simulink model "FOC_Motor_Control"  (R2020b)
settings: Solver=FixedStepDiscrete  StartTime=0.0  StopTime=10.0  FixedStep=Fixed_Step_Size  RelTol=1e-3
values from neighbouring files (symbols this model uses):
  Angle = 1.0    [Hall_Flux_FOC_Data.sldd]    (also in Motor_Control_Data.sldd)
  Cosine_table = 1.0 0.99999529 0.99999058 0.99998587 0.99998116 0.99996704 0.99995291 0.99993885 0.99992472 0.99990118 0.99987763 0.99985409 0.9998306 0.99979764 0.99976468 0.99973178 0.99969882 0.99965644 0.99961412 0.99957174 0.99952942 0.99947762 0.99942589 0.99937415 0.99932235 0.9992612 0.99920005 0.99913889 0.99907768 0.99900717 0.99893659 0.99886602 0.99879545 0.99871546 0.99863547 0.99855554 0.99847555 0.    [Hall_Flux_FOC_Data.sldd]    (also in Motor_Control_Data.sldd)
  Flux = 0.0109    [G474_FOC_LADRC.sldd]    (also in G474_FOC_NONOBSERVER.sldd = 0.0109
  HaLL_AngleShift = -0.25    [Hall_Flux_FOC_Data.sldd]
  HaLL_Sector1 = 5.236    [Hall_Flux_FOC_Data.sldd]
  HaLL_Sector2 = 1.0472    [Hall_Flux_FOC_Data.sldd]
  HaLL_Sector3 = 0.0    [Hall_Flux_FOC_Data.sldd]
  HaLL_Sector4 = 3.1415    [Hall_Flux_FOC_Data.sldd]
  HaLL_Sector5 = 4.1888    [Hall_Flux_FOC_Data.sldd]
  HaLL_Sector6 = 2.0944    [Hall_Flux_FOC_Data.sldd]
  HaLL_Timer_T = 1.0E-5    [Hall_Flux_FOC_Data.sldd]
  ID_Ki = 1.3    [Hall_Flux_FOC_Data.sldd]    (also in Motor_Control_Data.sldd = 48.0
  ID_Kp = 0.4    [Hall_Flux_FOC_Data.sldd]    (also in Motor_Control_Data.sldd = 0.84
  inverter = struct    [PMSM_Parameters.m]
  IQ_Ki = 1.6    [Hall_Flux_FOC_Data.sldd]    (also in Motor_Control_Data.sldd = 48.0
  IQ_Kp = 0.4    [Hall_Flux_FOC_Data.sldd]    (also in Motor_Control_Data.sldd = 1.869
  LADRC_b0 = 10000.0    [G474_FOC_LADRC.sldd]    (also in Hall_Flux_FOC_Data.sldd = 80000.0
  LADRC_Omega_c = 100.0    [G474_FOC_LADRC.sldd]    (also in Hall_Flux_FOC_Data.sldd = 80.0
  Ld = 0.0004    [Hall_Flux_FOC_Data.sldd]    (also in Motor_Control_Data.sldd = 0.00014
  Lq = 0.00045    [Hall_Flux_FOC_Data.sldd]    (also in Motor_Control_Data.sldd = 0.0003115
  OPL_Speed = 800.0    [Hall_Flux_FOC_Data.sldd]
  OPL_Time = 2.0    [Hall_Flux_FOC_Data.sldd]
  OPL_Torque = 3.0    [Hall_Flux_FOC_Data.sldd]
  Over_modulation = 0.0    [Hall_Flux_FOC_Data.sldd]    (also in Motor_Control_Data.sldd)
  pll_omega = 5000.0    [G474_FOC_LADRC.sldd]    (also in G474_FOC_NONOBSERVER.sldd)
  pll_xi = 10.0    [G474_FOC_LADRC.sldd]    (also in G474_FOC_NONOBSERVER.sldd)
  Pole_Pairs = 2.0    [Hall_Flux_FOC_Data.sldd]    (also in Motor_Control_Data.sldd = 4.0
  PWM_Frequency = 10000.0    [Hall_Flux_FOC_Data.sldd]    (also in Motor_Control_Data.sldd = 20000.0
  R = 0.405    [Hall_Flux_FOC_Data.sldd]    (also in Motor_Control_Data.sldd = 0.016
  Sine_table = 0.0 0.0015339879 0.0030679768 0.0046019657 0.0061359555 0.0076698866 0.0092038177 0.010737749 0.012271681 0.013805497 0.015339312 0.016873131 0.018406944 0.019940587 0.021474229 0.023007872 0.024541514 0.026074925 0.027608337 0.029141748 0.03067516 0.032208283 0.033741407 0.035274528 0.036807653 0.038340431 0.039873205 0.04140598 0.042938754 0.04447113 0.046003502 0.047535874 0.049068246 0.0506001    [Hall_Flux_FOC_Data.sldd]    (also in Motor_Control_Data.sldd)
  Speed_Ki = 0.06    [Hall_Flux_FOC_Data.sldd]    (also in Motor_Control_Data.sldd = 10.809
  Speed_Kp = 0.002    [Hall_Flux_FOC_Data.sldd]    (also in Motor_Control_Data.sldd = 0.08
  Speed_PI_OutputMax = 3.0    [Hall_Flux_FOC_Data.sldd]    (also in Motor_Control_Data.sldd = 700.0
  Speed_PI_OutputMin = -5.0    [Hall_Flux_FOC_Data.sldd]    (also in Motor_Control_Data.sldd = -700.0
  SpeedFilter_Fn = 0.3    [Hall_Flux_FOC_Data.sldd]    (also in Motor_Control_Data.sldd = 0.2
  TorqueMode = 0.0    [Hall_Flux_FOC_Data.sldd]    (also in Motor_Control_Data.sldd)
undefined symbols (not defined in the file or in its folder): DiscIntNeverNeededParam, Flux_Gain, Flux_Theta_Enable, magnitude, SVPWM
libraries: simulink x6, dspstat3 x1, pid_lib x1
(part 2 of 3)

== system FOC_Motor_Control/Motor_Control/Motor_Control_Function/FOC_Control_100us/FOC/Inverse_Park_Transform ==
  D : Inport
  Q : Inport  Port=2
  Sin_Coefficient : Inport  Port=3
  Cos_Coefficient : Inport  Port=4
  Theta : Inport  Port=5
  Add : Sum
  Add1 : Sum  Inputs=+-  OutDataTypeStr=Inherit: Same as first input
  Add2 : Sum  OutDataTypeStr=Inherit: Same as first input
  Add3 : Sum
  Cos_Coefficient1 : InportShadow  Port=4
  Harmonic_injection : Subsystem  Commented=on
  Product{1..4} (4 alike) : Product  RndMeth=Simplest  OutDataTypeStr=Inherit: Same as first input
  Scope : Scope  NumInputPorts=2
  Sin_Coefficient1 : InportShadow  Port=3
  Alpha : Outport  VectorParamsAs1DForOutWhenUnconnected=off
  Beta : Outport  Port=2  VectorParamsAs1DForOutWhenUnconnected=off
  wires:
  Product3/1 -> Add2/1
  Product4/1 -> Add2/2
  Product1/1 -> Add1/1
  Product2/1 -> Add1/2
  Cos_Coefficient1/1 -> Product4/2
  Sin_Coefficient/1 -> Product2/2
  D/1 -> Product3/1, Product1/1
  Q/1 -> Product2/1, Product4/1
  Sin_Coefficient1/1 -> Product3/2
  Cos_Coefficient/1 -> Product1/2
  Add1/1 -> Add/1
  Add/1 -> Alpha/1
  Harmonic_injection/1(Out1) -> Scope/1, Add/2
  Add2/1 -> Add3/2
  Add3/1 -> Beta/1
  Harmonic_injection/2(Out2) -> Scope/2, Add3/1
  Theta/1 -> Harmonic_injection/1(Input)

== system FOC_Motor_Control/Motor_Control/Motor_Control_Function/FOC_Control_100us/FOC/Obs_Angle ==
  Obs_Angle : Inport
  Action Port : ActionPort  ActionPortLabel=if(u1==1)
  Out1 : Outport
  wires:
  Obs_Angle/1 -> Out1/1

== system FOC_Motor_Control/Motor_Control/Motor_Control_Function/FOC_Control_100us/FOC/OpenLoop ==
  OPL_Speed : Inport
  OPL_Torque : Inport  Port=2
  OPL_Time : Inport  Port=3
  Action Port : ActionPort  ActionPortLabel=case [ 1 ]:
  2pi2 : Constant  Value=2*pi  OutDataTypeStr=single
  Discrete-Time Integrator1 : DiscreteIntegrator  SampleTime=-1  ICPrevOutput=DiscIntNeverNeededParam  ICPrevScaledInput=DiscIntNeverNeededParam
  Discrete-Time Integrator2 : DiscreteIntegrator  SampleTime=-1  ICPrevOutput=DiscIntNeverNeededParam  ICPrevScaledInput=DiscIntNeverNeededParam
  Mod2 : Math  Operator=mod  SaturateOnIntegerOverflow=on
  Product : Product
  Scope : Scope
  Scope1 : Scope
  We : Gain  Gain=Pole_Pairs*2*pi/60  OutDataTypeStr=single  ParamDataTypeStr=Inherit: Same as input
  Force_Angle : Outport
  OPL_Torque_Com : Outport  Port=2
  wires:
  OPL_Speed/1 -> Product/1
  Product/1 -> Discrete-Time Integrator2/1
  Discrete-Time Integrator1/1 -> Mod2/1
  Discrete-Time Integrator2/1 -> Scope/1, We/1
  We/1 -> Discrete-Time Integrator1/1  "Delta_Theta"
  Mod2/1 -> Force_Angle/1, Scope1/1
  OPL_Torque/1 -> OPL_Torque_Com/1
  OPL_Time/1 -> Product/2
  2pi2/1 -> Mod2/2

== system FOC_Motor_Control/Motor_Control/Motor_Control_Function/FOC_Control_100us/FOC/Park_Transform ==
  Alpha : Inport
  Beta : Inport  Port=2
  Sin_Coefficient : Inport  Port=3
  Cos_Coefficient : Inport  Port=4
  Add1 : Sum  OutDataTypeStr=Inherit: Same as first input
  Add2 : Sum  Inputs=-+  OutDataTypeStr=Inherit: Same as first input
  Alpha1 : InportShadow
  Beta1 : InportShadow  Port=2
  Cos_Coefficient1 : InportShadow  Port=4
  Produc3t : Product  RndMeth=Simplest  OutDataTypeStr=Inherit: Same as first input
  Product1 : Product  RndMeth=Simplest  OutDataTypeStr=Inherit: Same as first input
  Product2 : Product  RndMeth=Simplest  OutDataTypeStr=Inherit: Same as first input
  Product4 : Product  RndMeth=Simplest  OutDataTypeStr=Inherit: Same as first input
  Sin_Coefficient1 : InportShadow  Port=3
  D : Outport  VectorParamsAs1DForOutWhenUnconnected=off
  Q : Outport  Port=2  VectorParamsAs1DForOutWhenUnconnected=off
  wires:
  Produc3t/1 -> Add2/1
  Product4/1 -> Add2/2
  Product1/1 -> Add1/1
  Product2/1 -> Add1/2
  Alpha1/1 -> Produc3t/1
  Sin_Coefficient1/1 -> Produc3t/2
  Cos_Coefficient1/1 -> Product4/2
  Beta1/1 -> Product4/1
  Alpha/1 -> Product1/1
  Cos_Coefficient/1 -> Product1/2
  Beta/1 -> Product2/1
  Sin_Coefficient/1 -> Product2/2
  Add1/1 -> D/1
  Add2/1 -> Q/1

== system FOC_Motor_Control/Motor_Control/Motor_Control_Function/FOC_Control_100us/FOC/Q_Current_PI ==
  Reset : Inport
  Bus_voltage : Inport  Port=2
  Current_Command : Inport  Port=3
  Current_Measured : Inport  Port=4
  Add2 : Sum  Inputs=|+-
  IQ_Control : Subsystem
  Vq_voltage : Outport  VectorParamsAs1DForOutWhenUnconnected=off
  wires:
  Current_Command/1 -> Add2/1
  Current_Measured/1 -> Add2/2
  Add2/1 -> IQ_Control/3(Err)  "currentControlError"
  Reset/1 -> IQ_Control/1(Reset)
  Bus_voltage/1 -> IQ_Control/2(Bus_voltage)
  IQ_Control/1(PI_Out) -> Vq_voltage/1

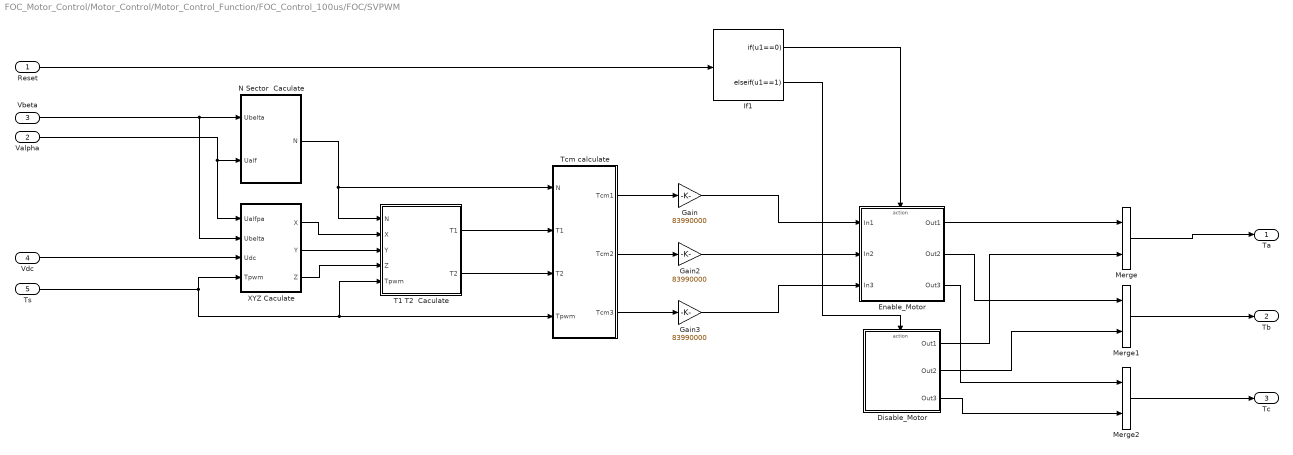
== system FOC_Motor_Control/Motor_Control/Motor_Control_Function/FOC_Control_100us/FOC/SVPWM ==
  Reset : Inport
  Valpha : Inport  Port=2
  Vbeta : Inport  Port=3
  Vdc : Inport  Port=4
  Ts : Inport  Port=5
  Disable_Motor : Subsystem  TreatAsAtomicUnit=on
  Enable_Motor : Subsystem  TreatAsAtomicUnit=on
  Gain : Gain  Gain=83990000
  Gain2 : Gain  Gain=83990000
  Gain3 : Gain  Gain=83990000
  If1 : If  IfExpression=u1==0  ElseIfExpressions=u1==1  ShowElse=off
  Merge : Merge
  Merge1 : Merge
  Merge2 : Merge
  N Sector  Caculate : Subsystem  TreatAsAtomicUnit=on
  T1 T2  Caculate : Subsystem  TreatAsAtomicUnit=on
  Tcm calculate : Subsystem  TreatAsAtomicUnit=on
  XYZ Caculate : Subsystem  TreatAsAtomicUnit=on
  Ta : Outport
  Tb : Outport  Port=2
  Tc : Outport  Port=3
  wires:
  T1 T2  Caculate/2(T2) -> Tcm calculate/3(T2)
  XYZ Caculate/1(X) -> T1 T2  Caculate/2(X)
  N Sector  Caculate/1(N) -> T1 T2  Caculate/1(N), Tcm calculate/1(N)
  Vdc/1 -> XYZ Caculate/3(Udc)
  T1 T2  Caculate/1(T1) -> Tcm calculate/2(T1)
  XYZ Caculate/3(Z) -> T1 T2  Caculate/4(Z)
  XYZ Caculate/2(Y) -> T1 T2  Caculate/3(Y)
  Valpha/1 -> N Sector  Caculate/2(Ualf), XYZ Caculate/1(Ualfpa)
  Vbeta/1 -> N Sector  Caculate/1(Ubelta), XYZ Caculate/2(Ubelta)
  Ts/1 -> T1 T2  Caculate/5(Tpwm), Tcm calculate/4(Tpwm), XYZ Caculate/4(Tpwm)
  Gain/1 -> Enable_Motor/1(In1)
  Gain2/1 -> Enable_Motor/2(In2)
  Reset/1 -> If1/1
  If1/1 -> Enable_Motor/Action
  If1/2 -> Disable_Motor/Action
  Gain3/1 -> Enable_Motor/3(In3)
  Enable_Motor/1(Out1) -> Merge/1
  Disable_Motor/1(Out1) -> Merge/2
  Enable_Motor/2(Out2) -> Merge1/1
  Disable_Motor/2(Out2) -> Merge1/2
  Enable_Motor/3(Out3) -> Merge2/1
  Disable_Motor/3(Out3) -> Merge2/2
  Merge/1 -> Ta/1
  Merge1/1 -> Tb/1
  Merge2/1 -> Tc/1
  Tcm calculate/1(Tcm1) -> Gain/1
  Tcm calculate/2(Tcm2) -> Gain2/1
  Tcm calculate/3(Tcm3) -> Gain3/1

== system FOC_Motor_Control/Motor_Control/Motor_Control_Function/FOC_Control_100us/FOC/Sine_Cosine ==
  note: Sine Cosine Coefficients
  P : Inport
  Cosine : Lookup_n-D  NumberOfTableDimensions=1  LookupTableObject=''  BreakpointsForDimension1=[0:2*pi/4095:2*pi]  BreakpointsForDimension1FirstPoint=10  BreakpointsForDimension2FirstPoint=10  BreakpointsForDimension1Spacing=12  BreakpointsForDimension2Spacing=12  IndexSearchMethod=Evenly spaced points  Table=Cosine_table  InterpMethod=Flat  DiagnosticForOutOfRangeInput=Error  InternalRulePriority=Speed  RndMeth=Simplest  InputSameDT=on
  Saturation : Saturate  UpperLimit=2*pi-0.0001  LowerLimit=0+0.0001
  Scope : Scope  NumInputPorts=2
  Sine : Lookup_n-D  NumberOfTableDimensions=1  LookupTableObject=''  BreakpointsForDimension1=[0:2*pi/4095:2*pi]  BreakpointsForDimension1FirstPoint=10  BreakpointsForDimension2FirstPoint=10  BreakpointsForDimension1Spacing=12  BreakpointsForDimension2Spacing=12  IndexSearchMethod=Evenly spaced points  Table=Sine_table  InterpMethod=Flat  DiagnosticForOutOfRangeInput=Error  InternalRulePriority=Speed  RndMeth=Simplest  InputSameDT=on
  Sin : Outport  VectorParamsAs1DForOutWhenUnconnected=off
  Cos : Outport  Port=2  VectorParamsAs1DForOutWhenUnconnected=off
  wires:
  P/1 -> Saturation/1  "position"
  Sine/1 -> Scope/1, Sin/1
  Cosine/1 -> Scope/2, Cos/1
  Saturation/1 -> Cosine/1, Sine/1

== system FOC_Motor_Control/Motor_Control/Motor_Control_Function/FOC_Control_100us/FOC/Subsystem ==
  In1 : Inport
  In2 : Inport  Port=2
  Action Port : ActionPort  ActionPortLabel=case [ 2 ]:
  Out1 : Outport
  Out2 : Outport  Port=2
  wires:
  In1/1 -> Out1/1
  In2/1 -> Out2/1

== system FOC_Motor_Control/Motor_Control/Motor_Control_Function/Angle_Speed_100us/SpeedAndAngle/ACC_OMG/LPF ==
  u : Inport
  Add : Sum  Inputs=+-
  Add1 : Sum
  Constant1 : Constant  Value=SpeedFilter_Fn  OutDataTypeStr=single
  Divide1 : Product  Inputs=**
  Unit Delay : UnitDelay  SampleTime=-1  HasFrameUpgradeWarning=on
  y : Outport
  wires:
  Constant1/1 -> Divide1/1
  u/1 -> Add/1
  Add/1 -> Divide1/2
  Divide1/1 -> Add1/1
  Unit Delay/1 -> Add/2, Add1/2
  Add1/1 -> Unit Delay/1, y/1

== system FOC_Motor_Control/Motor_Control/Motor_Control_Function/Angle_Speed_100us/SpeedAndAngle/ACC_OMG/Six_point ==
  In1 : Inport
  Merge2 : Merge  Inputs=6
  Scope : Scope  NumInputPorts=2
  Sector_1 : Subsystem
  Sector_2 : Subsystem
  Sector_3 : Subsystem
  Sector_4 : Subsystem
  Sector_5 : Subsystem
  Sector_6 : Subsystem
  Switch Case2 : SwitchCase  CaseConditions={1,2,3,4,5,6}  ShowDefaultCase=off
  Out1 : Outport
  wires:
  Sector_4/1(Angle_0) -> Merge2/4
  Switch Case2/5 -> Sector_5/Action
  Sector_6/1(Angle_0) -> Merge2/6
  Sector_5/1(Angle_0) -> Merge2/5
  Switch Case2/6 -> Sector_6/Action
  Switch Case2/3 -> Sector_3/Action
  Switch Case2/4 -> Sector_4/Action
  Sector_1/1(Angle_0) -> Merge2/1
  Switch Case2/2 -> Sector_2/Action
  In1/1 -> Scope/1, Switch Case2/1
  Sector_3/1(Angle_0) -> Merge2/3
  Switch Case2/1 -> Sector_1/Action
  Sector_2/1(Angle_0) -> Merge2/2
  Merge2/1 -> Scope/2, Out1/1

== system FOC_Motor_Control/Motor_Control/Motor_Control_Function/Angle_Speed_100us/SpeedAndAngle/ADC_IRQ/HallAngle_calibration ==
  Angle_input : Inport
  Angle_offset : Constant  Value=HaLL_AngleShift
  If Action Subsystem1 : Subsystem  TreatAsAtomicUnit=on
  If Action Subsystem2 : Subsystem  TreatAsAtomicUnit=on
  If Action Subsystem3 : Subsystem  TreatAsAtomicUnit=on
  If1 : If  IfExpression=u1 > 6.283185307  ElseIfExpressions=u1<0
  Merge1 : Merge  Inputs=3
  Subtract1 : Sum
  Angle_output : Outport
  wires:
  Angle_input/1 -> Subtract1/1
  Angle_offset/1 -> Subtract1/2  "Control_ModeCommand"
  If1/1 -> If Action Subsystem2/Action
  If1/3 -> If Action Subsystem1/Action
  If Action Subsystem2/1(Out1) -> Merge1/1
  Subtract1/1 -> If Action Subsystem3/1(In1), If Action Subsystem1/1(In1), If Action Subsystem2/1(In1), If1/1
  If Action Subsystem1/1(Out1) -> Merge1/3
  If Action Subsystem3/1(Out1) -> Merge1/2
  If1/2 -> If Action Subsystem3/Action
  Merge1/1 -> Angle_output/1

== system FOC_Motor_Control/Motor_Control/Motor_Control_Function/Angle_Speed_100us/Speed_Resolver/Speed_cacl/LPF ==
  u : Inport
  Add : Sum  Inputs=+-
  Add1 : Sum
  Constant1 : Constant  Value=SpeedFilter_Fn  OutDataTypeStr=single
  Divide1 : Product  Inputs=**
  Unit Delay : UnitDelay  SampleTime=-1  HasFrameUpgradeWarning=on
  y : Outport
  wires:
  Constant1/1 -> Divide1/1
  u/1 -> Add/1
  Add/1 -> Divide1/2
  Divide1/1 -> Add1/1
  Unit Delay/1 -> Add/2, Add1/2
  Add1/1 -> Unit Delay/1, y/1

== system FOC_Motor_Control/Motor_Control/Motor_Control_Function/Control_Command_2ms/Control_Command_2ms/Speed_PI/SpeedLoop ==
  CMD_RPM : Inport  OutDataTypeStr=single
  FdkRPM : Inport  Port=2  OutDataTypeStr=single
  Reset : Inport  Port=3
  Constant : Constant  Value=LADRC_b0  OutDataTypeStr=single  SampleTime=-1
  Divide : Product  Inputs=*/  OutDataTypeStr=single
  LESO : Subsystem
  Saturation : Saturate  UpperLimit=Speed_PI_OutputMax  LowerLimit=Speed_PI_OutputMin  OutDataTypeStr=single
  Sum : Sum  Inputs=|+-  OutDataTypeStr=single
  Sum1 : Sum  Inputs=|+-  OutDataTypeStr=single
  Unit Delay : UnitDelay  SampleTime=-1  HasFrameUpgradeWarning=on
  omega_c : Gain  Gain=LADRC_Omega_c  OutDataTypeStr=single
  RefIq : Outport  OutDataTypeStr=single
  wires:
  Saturation/1 -> RefIq/1, Unit Delay/1
  Constant/1 -> Divide/2
  Divide/1 -> Saturation/1
  LESO/2(f_hat) -> Sum1/2
  FdkRPM/1 -> LESO/1(FbkSpd)  "FdkRPM"
  LESO/1(omega_r_hat) -> Sum/2
  Sum1/1 -> Divide/1
  omega_c/1 -> Sum1/1
  Sum/1 -> omega_c/1
  CMD_RPM/1 -> Sum/1  "CMD_RPM"
  Unit Delay/1 -> LESO/2(iq)
  Reset/1 -> LESO/3(Reset)

== system FOC_Motor_Control/Motor_Control/Motor_Control_Function/Control_Command_2ms/Control_Command_2ms/Speed_PI/Speed_PI ==
  Ref : Inport
  Fdk : Inport  Port=2
  Reset : Inport  Port=3
  Speed_Control : Subsystem
  Sum : Sum  Inputs=|+-
  PI_out : Outport  VectorParamsAs1DForOutWhenUnconnected=off
  wires:
  Speed_Control/1(PI_Out) -> PI_out/1
  Reset/1 -> Speed_Control/2(Reset)
  Ref/1 -> Sum/1
  Sum/1 -> Speed_Control/1(Err)
  Fdk/1 -> Sum/2

== system FOC_Motor_Control/Motor_Control/Motor_Control_Function/FOC_Control_100us/FOC/Clarke_Transform/Clark1 ==
  Iabc : Inport
  Add : Sum  Inputs=+--
  Add1 : Sum  Inputs=+-
  Demux : Demux  Outputs=3
  Gain : Gain  Gain=0.5
  Gain1 : Gain  Gain=0.5
  Gain2 : Gain  Gain=sqrt(2/3)
  Gain3 : Gain  Gain=sqrt(3)/2
  Gain4 : Gain  Gain=sqrt(3)/2
  Gain5 : Gain  Gain=sqrt(2/3)
  Ialpha : Outport  VectorParamsAs1DForOutWhenUnconnected=off
  Ibeta : Outport  Port=2  VectorParamsAs1DForOutWhenUnconnected=off
  wires:
  Iabc/1 -> Demux/1
  Demux/1 -> Add/1
  Gain/1 -> Add/2
  Demux/2 -> Gain3/1, Gain/1
  Gain1/1 -> Add/3
  Demux/3 -> Gain4/1, Gain1/1
  Add/1 -> Gain2/1
  Gain2/1 -> Ialpha/1
  Gain3/1 -> Add1/1
  Gain4/1 -> Add1/2
  Add1/1 -> Gain5/1
  Gain5/1 -> Ibeta/1

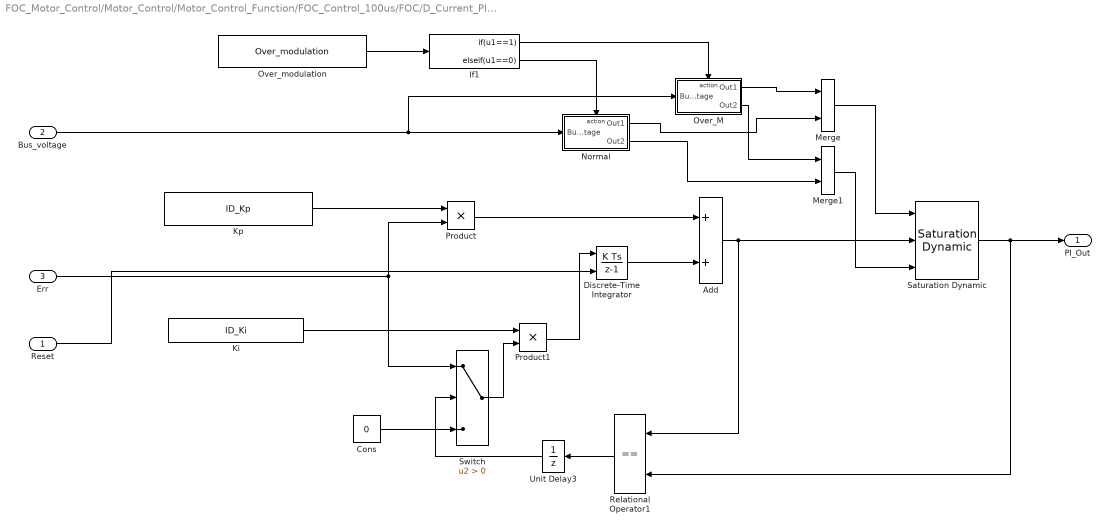
== system FOC_Motor_Control/Motor_Control/Motor_Control_Function/FOC_Control_100us/FOC/D_Current_PI/ID_Control ==
  Reset : Inport
  Bus_voltage : Inport  Port=2
  Err : Inport  Port=3
  Add : Sum
  Cons : Constant  Value=0  OutDataTypeStr=single
  Discrete-Time Integrator : DiscreteIntegrator  ExternalReset=level  SampleTime=-1  ICPrevOutput=DiscIntNeverNeededParam  ICPrevScaledInput=DiscIntNeverNeededParam
  If1 : If  IfExpression=u1==1  ElseIfExpressions=u1==0  ShowElse=off
  Ki : Constant  Value=ID_Ki  OutDataTypeStr=single
  Kp : Constant  Value=ID_Kp  OutDataTypeStr=single
  Merge : Merge
  Merge1 : Merge
  Normal : Subsystem  TreatAsAtomicUnit=on
  Over_M : Subsystem  TreatAsAtomicUnit=on
  Over_modulation : Constant  Value=Over_modulation  OutDataTypeStr=boolean
  Product : Product
  Product1 : Product
  Relational Operator1 : RelationalOperator  Operator===  OutDataTypeStr=boolean  RndMeth=Simplest
  Saturation Dynamic : simulink/Discontinuities/Saturation Dynamic  OutMin=[]  OutMax=[]  OutDataTypeStr=Inherit: Same as second input  OutDataType=fixdt(1, 16)  OutScaling=2^-10  DoSatur=off
  Switch : Switch  Criteria=u2 > Threshold
  Unit Delay3 : UnitDelay  SampleTime=-1  HasFrameUpgradeWarning=on
  PI_Out : Outport
  wires:
  Kp/1 -> Product/1
  Err/1 -> Product/2, Switch/1
  Switch/1 -> Product1/2
  Product1/1 -> Discrete-Time Integrator/1
  Product/1 -> Add/1
  Add/1 -> Saturation Dynamic/2, Relational Operator1/1
  Saturation Dynamic/1 -> Relational Operator1/2, PI_Out/1
  Cons/1 -> Switch/3
  Discrete-Time Integrator/1 -> Add/2
  Relational Operator1/1 -> Unit Delay3/1
  Ki/1 -> Product1/1
  Unit Delay3/1 -> Switch/2
  Reset/1 -> Discrete-Time Integrator/2
  Over_modulation/1 -> If1/1
  If1/2 -> Normal/Action
  If1/1 -> Over_M/Action
  Bus_voltage/1 -> Over_M/1(Bus_voltage), Normal/1(Bus_voltage)
  Over_M/1(Out1) -> Merge/1
  Normal/1(Out1) -> Merge/2
  Over_M/2(Out2) -> Merge1/1
  Normal/2(Out2) -> Merge1/2
  Merge/1 -> Saturation Dynamic/1
  Merge1/1 -> Saturation Dynamic/3

== system FOC_Motor_Control/Motor_Control/Motor_Control_Function/FOC_Control_100us/FOC/Flux_Observer/OBSERVER ==
  i_alpha : Inport  OutDataTypeStr=single
  i_beta : Inport  Port=2  OutDataTypeStr=single
  u_alpha : Inport  Port=3  OutDataTypeStr=single
  u_beta : Inport  Port=4  OutDataTypeStr=single
  Abs : Abs  OutDataTypeStr=single
  Atan2 : Trigonometry  Operator=atan2
  Cacl_X1X2_Hat : Subsystem
  Cacl_Y1Y2 : Subsystem
  Constant : Constant  Value=2*pi  OutDataTypeStr=single
  Gain1 : Gain  Gain=15/pi
  LPF : Subsystem
  Mod : Math  Operator=mod  SaturateOnIntegerOverflow=on
  Moving Average : dspstat3/Moving Average  Method=Exponential weighting  ForgettingFactorPort=off  SpecifyWindowLength=on  WindowLength=4  ForgettingFactor=0.99  SimulateUsing=Code generation
  PLL : Subsystem
  Terminator : Terminator
  Obs_Theta : Outport
  Obs_Speed : Outport  Port=2
  wires:
  i_beta/1 -> Cacl_X1X2_Hat/4(i_beta), Cacl_Y1Y2/3(i_beta)
  i_alpha/1 -> Cacl_X1X2_Hat/3(i_alpha), Cacl_Y1Y2/1(i_alpha)
  u_alpha/1 -> Cacl_Y1Y2/2(u_alpha)
  u_beta/1 -> Cacl_Y1Y2/4(u_beta)
  Cacl_Y1Y2/1(y1) -> Cacl_X1X2_Hat/1(y1)
  Cacl_Y1Y2/2(y2) -> Cacl_X1X2_Hat/2(y2)
  Abs/1 -> Moving Average/1
  Moving Average/1 -> Cacl_X1X2_Hat/5(omega_e_hat), Cacl_Y1Y2/5(omega_e_hat)
  PLL/1(Obs_Theta) -> Obs_Theta/1  "Obs_Theta"
  PLL/2(omega_e_hat) -> Gain1/1, Abs/1
  Gain1/1 -> LPF/1(u)
  LPF/1(y) -> Obs_Speed/1
  Atan2/1 -> Mod/1
  Cacl_X1X2_Hat/2(eta_x2_hat) -> Atan2/1, PLL/2(eta_x2_hat)
  Mod/1 -> Terminator/1  "atan2_Theata"
  Cacl_X1X2_Hat/1(eta_x1_hat) -> Atan2/2, PLL/1(eta_x1_hat)
  Constant/1 -> Mod/2

== system FOC_Motor_Control/Motor_Control/Motor_Control_Function/FOC_Control_100us/FOC/Inverse_Park_Transform/Harmonic_injection ==
  Input : Inport
  Gain2 : Gain  Gain=20
  Gain3 : Gain  Gain=-5
  Gain4 : Gain  Gain=20
  Gain5 : Gain  Gain=-5
  Gain6 : Gain  Gain=5
  Gain7 : Gain  Gain=7
  Gain8 : Gain  Gain=5
  Gain9 : Gain  Gain=7
  Sum3 : Sum  Inputs=|++
  Sum4 : Sum  Inputs=|++
  Trigonometric Function : Trigonometry  Operator=cos
  Trigonometric Function1 : Trigonometry
  Trigonometric Function2 : Trigonometry  Operator=cos
  Trigonometric Function3 : Trigonometry
  Out1 : Outport
  Out2 : Outport  Port=2
  wires:
  Trigonometric Function1/1 -> Gain4/1
  Trigonometric Function/1 -> Gain2/1
  Gain5/1 -> Trigonometric Function1/1
  Trigonometric Function2/1 -> Gain6/1
  Gain7/1 -> Trigonometric Function2/1
  Gain9/1 -> Trigonometric Function3/1
  Trigonometric Function3/1 -> Gain8/1
  Gain2/1 -> Sum3/1
  Gain3/1 -> Trigonometric Function/1
  Gain4/1 -> Sum4/1
  Gain6/1 -> Sum3/2
  Gain8/1 -> Sum4/2
  Sum3/1 -> Out1/1
  Sum4/1 -> Out2/1
  Input/1 -> Gain9/1, Gain5/1, Gain3/1, Gain7/1

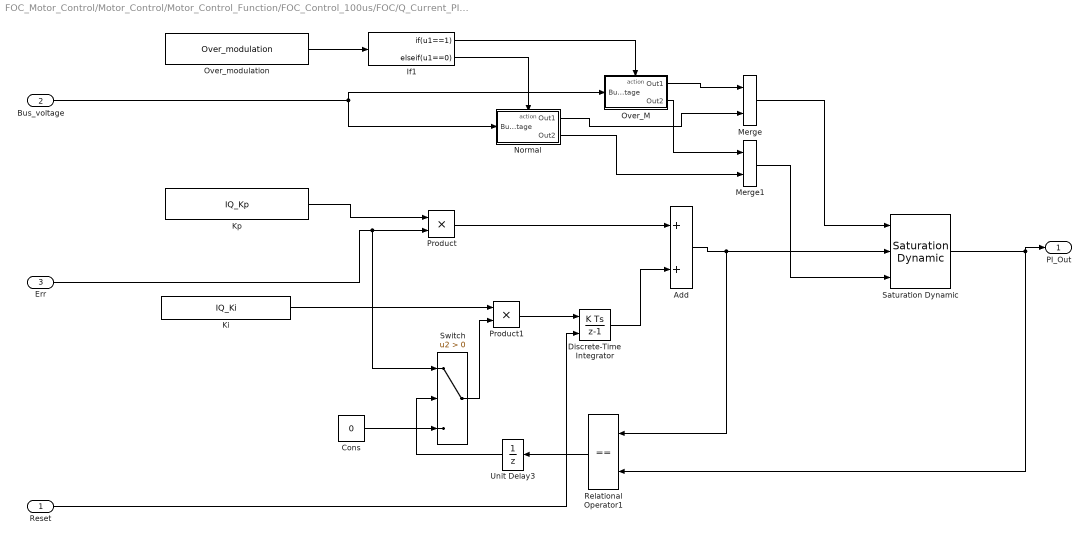
== system FOC_Motor_Control/Motor_Control/Motor_Control_Function/FOC_Control_100us/FOC/Q_Current_PI/IQ_Control ==
  Reset : Inport
  Bus_voltage : Inport  Port=2
  Err : Inport  Port=3
  Add : Sum
  Cons : Constant  Value=0  OutDataTypeStr=single
  Discrete-Time Integrator : DiscreteIntegrator  ExternalReset=level  SampleTime=-1  ICPrevOutput=DiscIntNeverNeededParam  ICPrevScaledInput=DiscIntNeverNeededParam
  If1 : If  IfExpression=u1==1  ElseIfExpressions=u1==0  ShowElse=off
  Ki : Constant  Value=IQ_Ki  OutDataTypeStr=single
  Kp : Constant  Value=IQ_Kp  OutDataTypeStr=single
  Merge : Merge
  Merge1 : Merge
  Normal : Subsystem  TreatAsAtomicUnit=on
  Over_M : Subsystem  TreatAsAtomicUnit=on
  Over_modulation : Constant  Value=Over_modulation  OutDataTypeStr=boolean
  Product : Product
  Product1 : Product
  Relational Operator1 : RelationalOperator  Operator===  OutDataTypeStr=boolean  RndMeth=Simplest
  Saturation Dynamic : simulink/Discontinuities/Saturation Dynamic  OutMin=[]  OutMax=[]  OutDataTypeStr=Inherit: Same as second input  OutDataType=fixdt(1, 16)  OutScaling=2^-10  DoSatur=off
  Switch : Switch  Criteria=u2 > Threshold
  Unit Delay3 : UnitDelay  SampleTime=-1  HasFrameUpgradeWarning=on
  PI_Out : Outport
  wires:
  Kp/1 -> Product/1
  Err/1 -> Switch/1, Product/2
  Switch/1 -> Product1/2
  Product1/1 -> Discrete-Time Integrator/1
  Product/1 -> Add/1
  Add/1 -> Saturation Dynamic/2, Relational Operator1/1
  Saturation Dynamic/1 -> PI_Out/1, Relational Operator1/2
  Cons/1 -> Switch/3
  Discrete-Time Integrator/1 -> Add/2
  Relational Operator1/1 -> Unit Delay3/1
  Ki/1 -> Product1/1
  Unit Delay3/1 -> Switch/2
  Reset/1 -> Discrete-Time Integrator/2
  Normal/1(Out1) -> Merge/2
  Over_M/1(Out1) -> Merge/1
  Over_modulation/1 -> If1/1
  Normal/2(Out2) -> Merge1/2
  If1/2 -> Normal/Action
  Bus_voltage/1 -> Normal/1(Bus_voltage), Over_M/1(Bus_voltage)
  If1/1 -> Over_M/Action
  Over_M/2(Out2) -> Merge1/1
  Merge/1 -> Saturation Dynamic/1
  Merge1/1 -> Saturation Dynamic/3

== system FOC_Motor_Control/Motor_Control/Motor_Control_Function/FOC_Control_100us/FOC/SVPWM/Disable_Motor ==
  Action Port : ActionPort  ActionPortLabel=elseif(u1==1)
  Constant : Constant  Value=0  OutDataTypeStr=single
  Constant1 : Constant  Value=0  OutDataTypeStr=single
  Constant2 : Constant  Value=0  OutDataTypeStr=single
  Out1 : Outport
  Out2 : Outport  Port=2
  Out3 : Outport  Port=3
  wires:
  Constant/1 -> Out1/1
  Constant1/1 -> Out2/1
  Constant2/1 -> Out3/1

== system FOC_Motor_Control/Motor_Control/Motor_Control_Function/FOC_Control_100us/FOC/SVPWM/Enable_Motor ==
  In1 : Inport
  In2 : Inport  Port=2
  In3 : Inport  Port=3
  Action Port : ActionPort  ActionPortLabel=if(u1==0)
  Saturation : Saturate  UpperLimit=4199  LowerLimit=1
  Saturation1 : Saturate  UpperLimit=4199  LowerLimit=1
  Saturation2 : Saturate  UpperLimit=4199  LowerLimit=1
  Out1 : Outport
  Out2 : Outport  Port=2
  Out3 : Outport  Port=3
  wires:
  In1/1 -> Saturation/1
  In2/1 -> Saturation1/1
  In3/1 -> Saturation2/1
  Saturation/1 -> Out1/1
  Saturation1/1 -> Out2/1
  Saturation2/1 -> Out3/1

== system FOC_Motor_Control/Motor_Control/Motor_Control_Function/FOC_Control_100us/FOC/SVPWM/N Sector  Caculate ==
  Ubelta : Inport
  Ualf : Inport  Port=2
  Add : Sum  Inputs=+++
  Add1 : Sum  Inputs=-+
  Add2 : Sum  Inputs=--
  Constant : Constant  OutDataTypeStr=single
  Constant1 : Constant  Value=0  OutDataTypeStr=single
  Gain : Gain  Gain=sqrt(3)
  Gain1 : Gain  Gain=2
  Gain2 : Gain  Gain=4
  Saturation : Saturate  UpperLimit=6  LowerLimit=1
  Switch : Switch
  Switch1 : Switch
  Switch2 : Switch
  N : Outport
  wires:
  Saturation/1 -> N/1
  Add/1 -> Saturation/1
  Gain2/1 -> Add/3
  Switch2/1 -> Gain2/1
  Add2/1 -> Switch2/2
  Gain1/1 -> Add/2
  Switch1/1 -> Gain1/1
  Add1/1 -> Switch1/2
  Gain/1 -> Add2/2, Add1/2
  Ualf/1 -> Gain/1
  Switch/1 -> Add/1
  Constant1/1 -> Switch/3, Switch1/3, Switch2/3
  Constant/1 -> Switch/1, Switch1/1, Switch2/1
  Ubelta/1 -> Add2/1, Add1/1, Switch/2

== system FOC_Motor_Control/Motor_Control/Motor_Control_Function/FOC_Control_100us/FOC/SVPWM/T1 T2  Caculate ==
  note: Z
  note: Y
  note: -X
  note: X
  note: -Y
  note: Y
  note: -X
  note: X
  note: Z
  note: -Y
  note: -Z
  note: X
  note: Y
  note: Z
  N : Inport
  X : Inport  Port=2
  Y : Inport  Port=3
  Z : Inport  Port=4
  Tpwm : Inport  Port=5
  Add : Sum
  Add1 : Sum  Inputs=-+
  Divide : Product  Inputs=**/
  Divide1 : Product  Inputs=/**
  Gain : Gain  Gain=-1
  Gain1 : Gain  Gain=-1
  Gain2 : Gain  Gain=-1
  Index Vector : MultiPortSwitch  Inputs=6
  Index Vector1 : MultiPortSwitch  Inputs=6
  Switch : Switch  Criteria=u2 > Threshold
  Switch2 : Switch  Criteria=u2 > Threshold
  T1 : Outport
  T2 : Outport  Port=2
  wires:
  Switch2/1 -> T2/1
  Divide1/1 -> Switch2/3
  Switch/1 -> T1/1
  Add1/1 -> Switch/2, Switch2/2
  Add/1 -> Divide1/1, Divide/3, Add1/1
  Tpwm/1 -> Divide1/2, Divide/2, Add1/2
  Divide/1 -> Switch/3
  Index Vector1/1 -> Switch2/1, Add/2, Divide1/3
  Index Vector/1 -> Switch/1, Divide/1, Add/1
  Gain1/1 -> Index Vector/7, Index Vector1/6
  Gain2/1 -> Index Vector/4, Index Vector1/7  "-Z"
  Gain/1 -> Index Vector/5, Index Vector1/3
  Y/1 -> Gain1/1, Index Vector/3, Index Vector1/2
  X/1 -> Index Vector1/4, Index Vector/6, Gain/1
  Z/1 -> Index Vector/2, Index Vector1/5, Gain2/1
  N/1 -> Index Vector1/1, Index Vector/1

== system FOC_Motor_Control/Motor_Control/Motor_Control_Function/FOC_Control_100us/FOC/SVPWM/Tcm calculate ==
  note: Tc
  note: Tb
  note: Ta
  N : Inport
  T1 : Inport  Port=2
  T2 : Inport  Port=3
  Tpwm : Inport  Port=4
  Add : Sum  Inputs=--+
  Add1 : Sum
  Add2 : Sum
  Gain : Gain  Gain=0.5
  Gain1 : Gain  Gain=0.5
  Gain2 : Gain  Gain=1/4
  Index Vector : MultiPortSwitch  Inputs=6
  Index Vector1 : MultiPortSwitch  Inputs=6
  Index Vector2 : MultiPortSwitch  Inputs=6
  Scope2 : Scope  NumInputPorts=3
  Tcm1 : Outport
  Tcm2 : Outport  Port=2
  Tcm3 : Outport  Port=3
  wires:
  Index Vector2/1 -> Scope2/3, Tcm3/1
  N/1 -> Index Vector/1, Index Vector1/1, Index Vector2/1
  Add2/1 -> Index Vector/5, Index Vector/6, Index Vector1/3, Index Vector1/7, Index Vector2/2, Index Vector2/4
  Gain1/1 -> Add2/1
  Add1/1 -> Add2/2, Index Vector/2, Index Vector/7, Index Vector1/4, Index Vector1/5, Index Vector2/3, Index Vector2/6
  Gain2/1 -> Index Vector2/5, Index Vector2/7, Add1/2, Index Vector/3, Index Vector/4, Index Vector1/2, Index Vector1/6
  Gain/1 -> Add1/1
  Add/1 -> Gain2/1
  Tpwm/1 -> Add/3
  T2/1 -> Add/2, Gain1/1
  T1/1 -> Add/1, Gain/1
  Index Vector/1 -> Scope2/1, Tcm1/1
  Index Vector1/1 -> Scope2/2, Tcm2/1

== system FOC_Motor_Control/Motor_Control/Motor_Control_Function/FOC_Control_100us/FOC/SVPWM/XYZ Caculate ==
  note: X
  note: Y
  note: Z
  Ualfpa : Inport
  Ubelta : Inport  Port=2
  Udc : Inport  Port=3
  Tpwm : Inport  Port=4
  Add1 : Sum  Inputs=-+
  Add2 : Sum  Inputs=--
  Constant : Constant  Value=sqrt(3)  OutDataTypeStr=single
  Divide : Product  Inputs=**/
  Gain : Gain  Gain=sqrt(3)
  Gain1 : Gain  Gain=-0.5
  Gain2 : Gain  Gain=-0.5
  Product : Product
  Product1 : Product
  Product2 : Product
  Saturation : Saturate  UpperLimit=1200  LowerLimit=0.0001
  X : Outport
  Y : Outport  Port=2
  Z : Outport  Port=3
  wires:
  Gain2/1 -> Product1/1
  Add2/1 -> Gain2/1
  Add1/1 -> Gain1/1
  Gain/1 -> Add2/2, Add1/2
  Ualfpa/1 -> Gain/1
  Ubelta/1 -> Add2/1, Add1/1, Product/1
  Gain1/1 -> Product2/2
  Product2/1 -> Z/1
  Divide/1 -> Product1/2, Product2/1, Product/2
  Product1/1 -> Y/1
  Product/1 -> X/1
  Udc/1 -> Saturation/1
  Tpwm/1 -> Divide/2
  Constant/1 -> Divide/1
  Saturation/1 -> Divide/3

== system FOC_Motor_Control/Motor_Control/Motor_Control_Function/Angle_Speed_100us/SpeedAndAngle/ACC_OMG/Six_point/Sector_1 ==
  Action Port : ActionPort  ActionPortLabel=case [ 1 ]:
  Add : Sum
  Constant : Constant  Value=HaLL_Sector1  OutDataTypeStr=single
  Constant1 : Constant  Value=HaLL_AngleShift  OutDataTypeStr=single
  Angle_0 : Outport
  wires:
  Constant/1 -> Add/1
  Constant1/1 -> Add/2
  Add/1 -> Angle_0/1

== system FOC_Motor_Control/Motor_Control/Motor_Control_Function/Angle_Speed_100us/SpeedAndAngle/ACC_OMG/Six_point/Sector_2 ==
  Action Port : ActionPort  ActionPortLabel=case [ 2 ]:
  Add : Sum
  Constant1 : Constant  Value=HaLL_AngleShift  OutDataTypeStr=single
  Pi/3 : Constant  Value=HaLL_Sector2  OutDataTypeStr=single
  Angle_0 : Outport
  wires:
  Pi/3/1 -> Add/1
  Constant1/1 -> Add/2
  Add/1 -> Angle_0/1

== system FOC_Motor_Control/Motor_Control/Motor_Control_Function/Angle_Speed_100us/SpeedAndAngle/ACC_OMG/Six_point/Sector_3 ==
  Action Port : ActionPort  ActionPortLabel=case [ 3 ]:
  Add : Sum
  Constant : Constant  Value=HaLL_Sector3  OutDataTypeStr=single
  Constant1 : Constant  Value=HaLL_AngleShift  OutDataTypeStr=single
  Angle_0 : Outport
  wires:
  Constant/1 -> Add/1
  Add/1 -> Angle_0/1
  Constant1/1 -> Add/2

== system FOC_Motor_Control/Motor_Control/Motor_Control_Function/Angle_Speed_100us/SpeedAndAngle/ACC_OMG/Six_point/Sector_4 ==
  Action Port : ActionPort  ActionPortLabel=case [ 4 ]:
  Add : Sum
  Constant : Constant  Value=HaLL_Sector4  OutDataTypeStr=single
  Constant1 : Constant  Value=HaLL_AngleShift  OutDataTypeStr=single
  Angle_0 : Outport
  wires:
  Constant/1 -> Add/1
  Add/1 -> Angle_0/1
  Constant1/1 -> Add/2

== system FOC_Motor_Control/Motor_Control/Motor_Control_Function/Angle_Speed_100us/SpeedAndAngle/ACC_OMG/Six_point/Sector_5 ==
  Action Port : ActionPort  ActionPortLabel=case [ 5 ]:
  Add : Sum
  Constant : Constant  Value=HaLL_Sector5  OutDataTypeStr=single
  Constant1 : Constant  Value=HaLL_AngleShift  OutDataTypeStr=single
  Angle_0 : Outport
  wires:
  Constant/1 -> Add/1
  Add/1 -> Angle_0/1
  Constant1/1 -> Add/2

== system FOC_Motor_Control/Motor_Control/Motor_Control_Function/Angle_Speed_100us/SpeedAndAngle/ACC_OMG/Six_point/Sector_6 ==
  Action Port : ActionPort  ActionPortLabel=case [ 6 ]:
  Add : Sum
  Constant : Constant  Value=HaLL_Sector6  OutDataTypeStr=single
  Constant1 : Constant  Value=HaLL_AngleShift  OutDataTypeStr=single
  Angle_0 : Outport
  wires:
  Constant/1 -> Add/1
  Add/1 -> Angle_0/1
  Constant1/1 -> Add/2

== system FOC_Motor_Control/Motor_Control/Motor_Control_Function/Angle_Speed_100us/SpeedAndAngle/ADC_IRQ/HallAngle_calibration/If Action Subsystem1 ==
  In1 : Inport
  Action Port : ActionPort  ActionPortLabel=else
  Out1 : Outport
  wires:
  In1/1 -> Out1/1

== system FOC_Motor_Control/Motor_Control/Motor_Control_Function/Angle_Speed_100us/SpeedAndAngle/ADC_IRQ/HallAngle_calibration/If Action Subsystem2 ==
  In1 : Inport
  Action Port : ActionPort  ActionPortLabel=if(u1 > 6.283185307)
  2pi : Constant  Value=2*pi  OutDataTypeStr=single
  Subtract1 : Sum  Inputs=+-  OutDataTypeStr=single
  Out1 : Outport
  wires:
  In1/1 -> Subtract1/1
  Subtract1/1 -> Out1/1
  2pi/1 -> Subtract1/2

== system FOC_Motor_Control/Motor_Control/Motor_Control_Function/Angle_Speed_100us/SpeedAndAngle/ADC_IRQ/HallAngle_calibration/If Action Subsystem3 ==
  In1 : Inport
  Action Port : ActionPort  ActionPortLabel=elseif(u1<0)
  Angle_offset : Constant  Value=2*pi  OutDataTypeStr=single
  Subtract1 : Sum
  Out1 : Outport
  wires:
  In1/1 -> Subtract1/1
  Subtract1/1 -> Out1/1
  Angle_offset/1 -> Subtract1/2

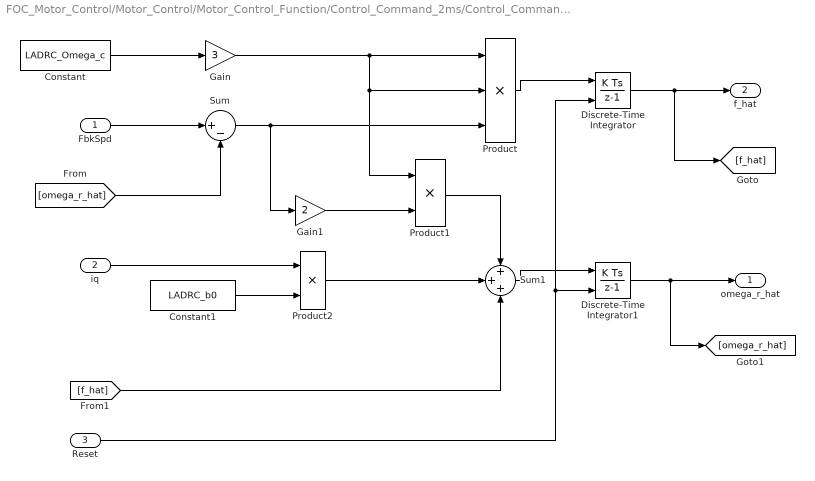
== system FOC_Motor_Control/Motor_Control/Motor_Control_Function/Control_Command_2ms/Control_Command_2ms/Speed_PI/SpeedLoop/LESO ==
  FbkSpd : Inport  OutDataTypeStr=single  PortDimensions=1
  iq : Inport  Port=2  OutDataTypeStr=single  PortDimensions=1
  Reset : Inport  Port=3
  Constant : Constant  Value=LADRC_Omega_c  OutDataTypeStr=single
  Constant1 : Constant  Value=LADRC_b0  OutDataTypeStr=single  SampleTime=-1
  Discrete-Time Integrator : DiscreteIntegrator  ExternalReset=level  SampleTime=-1  OutDataTypeStr=single  UpperSaturationLimit=6e4  LowerSaturationLimit=-6e4  ICPrevOutput=DiscIntNeverNeededParam  ICPrevScaledInput=DiscIntNeverNeededParam
  Discrete-Time Integrator1 : DiscreteIntegrator  ExternalReset=level  SampleTime=-1  OutDataTypeStr=single  LimitOutput=on  UpperSaturationLimit=2000  LowerSaturationLimit=-2000  ICPrevOutput=DiscIntNeverNeededParam  ICPrevScaledInput=DiscIntNeverNeededParam
  Gain : Gain  Gain=3  OutDataTypeStr=single
  Gain1 : Gain  Gain=2  OutDataTypeStr=single
  Product : Product  Inputs=3  OutDataTypeStr=single
  Product1 : Product  OutDataTypeStr=single
  Product2 : Product  OutDataTypeStr=single
  Sum : Sum  Inputs=|+-  OutDataTypeStr=single
  Sum1 : Sum  Inputs=+++  OutDataTypeStr=single
  omega_r_hat : Outport  OutDataTypeStr=single
  f_hat : Outport  Port=2  OutDataTypeStr=single
  wires:
  Sum/1 -> Gain1/1, Product/3
  Product/1 -> Discrete-Time Integrator/1
  Discrete-Time Integrator/1 -> [f_hat], f_hat/1
  [f_hat] -> Sum1/3
  Sum1/1 -> Discrete-Time Integrator1/1
  Discrete-Time Integrator1/1 -> omega_r_hat/1, [omega_r_hat]
  Product1/1 -> Sum1/1
  FbkSpd/1 -> Sum/1
  [omega_r_hat] -> Sum/2
  Constant/1 -> Gain/1
  Gain1/1 -> Product1/2
  Gain/1 -> Product1/1, Product/2, Product/1
  iq/1 -> Product2/1
  Constant1/1 -> Product2/2
  Product2/1 -> Sum1/2
  Reset/1 -> Discrete-Time Integrator/2, Discrete-Time Integrator1/2
